simulink model "car_linear_force"  (R2024b)
settings: Solver=VariableStepAuto  StartTime=0.0  StopTime=1  RelTol=1e-3
values from neighbouring files (symbols this model uses):
  Cd = [0 1]    [mpc3.m]
  Cr = 87342    [mpc3.m]    (also in prueba_mpc.m; prueba_mpc2.m)
  m = 1400    [mpc3.m]    (also in prueba_mpc.m; prueba_mpc2.m)
  R = 1    [prueba_mpc.m]    (also in prueba_mpc2.m)
undefined symbols (not defined in the file or in its folder): Af, C_lambda, g, mode, omega, theta
settings Model: Creator=inaki  LastModifiedBy=inaki

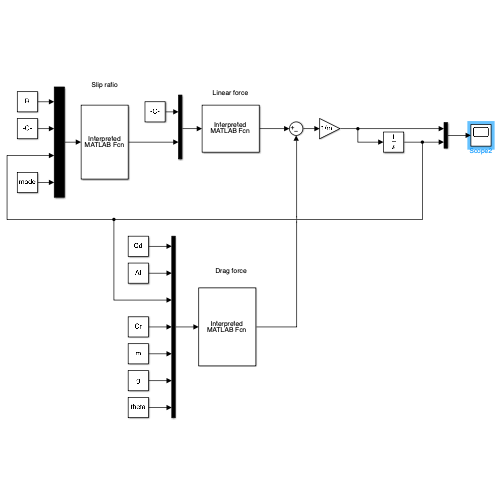
[thumbnail: Simulink's stored preview of the top-level diagram]
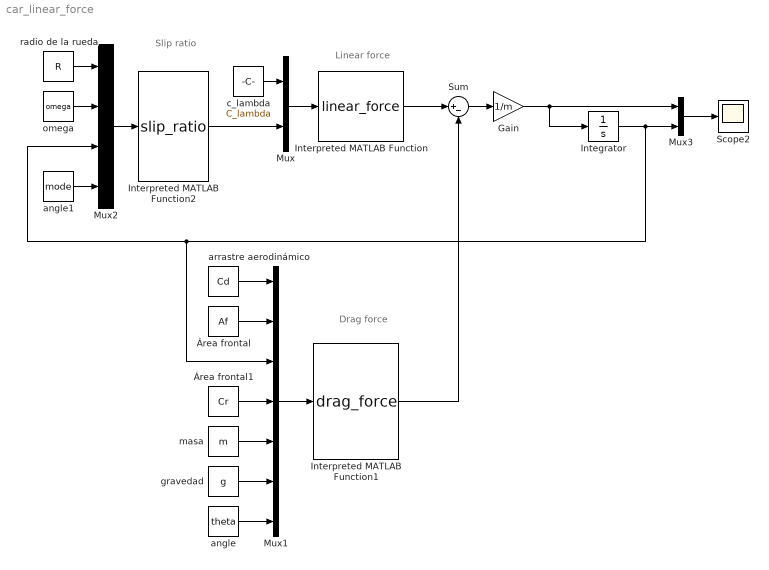
== system car_linear_force ==
  note: Drag force
  note: Linear force
  note: Slip ratio
  Gain : Gain  Gain=1/m
  Integrator : Integrator
  Interpreted MATLAB Function : MATLABFcn  MATLABFcn=linear_force  Output1D=off
  Interpreted MATLAB Function1 : MATLABFcn  MATLABFcn=drag_force  Output1D=off
  Interpreted MATLAB Function2 : MATLABFcn  MATLABFcn=slip_ratio  Output1D=off
  Mux : Mux  Inputs=2
  Mux1 : Mux  Inputs=7
  Mux2 : Mux
  Mux3 : Mux  Inputs=2
  Scope2 : Scope
  Sum : Sum  Inputs=|+-
  angle : Constant  Value=theta  VectorParams1D=off
  angle1 : Constant  Value=mode
  arrastre aerodinámico : Constant  Value=Cd  VectorParams1D=off
  c_lambda : Constant  Value=C_lambda
  gravedad : Constant  Value=g  VectorParams1D=off
  masa : Constant  Value=m  VectorParams1D=off
  omega : Constant  Value=omega  VectorParams1D=off
  radio de la rueda : Constant  Value=R  VectorParams1D=off
  Área frontal : Constant  Value=Af  VectorParams1D=off
  Área frontal1 : Constant  Value=Cr  VectorParams1D=off
  wires:
  Interpreted MATLAB Function2/1 -> Mux/2
  Área frontal/1 -> Mux1/2
  Área frontal1/1 -> Mux1/4
  masa/1 -> Mux1/5
  gravedad/1 -> Mux1/6
  angle/1 -> Mux1/7
  Mux1/1 -> Interpreted MATLAB Function1/1
  Interpreted MATLAB Function1/1 -> Sum/2
  radio de la rueda/1 -> Mux2/1
  omega/1 -> Mux2/2
  angle1/1 -> Mux2/4
  Sum/1 -> Gain/1
  Gain/1 -> Mux3/1, Integrator/1
  Mux3/1 -> Scope2/1
  Mux2/1 -> Interpreted MATLAB Function2/1
  c_lambda/1 -> Mux/1
  Mux/1 -> Interpreted MATLAB Function/1
  Interpreted MATLAB Function/1 -> Sum/1
  Integrator/1 -> Mux3/2, Mux2/3, Mux1/3
  arrastre aerodinámico/1 -> Mux1/1
